simulink model "part2_2"  (R2018b)
settings: Solver=VariableStepAuto  StartTime=0.0  StopTime=10.0*0.1551  MaxStep=0.01*0.1551  RelTol=1e-3
settings Model: Creator=buddyugwumba1  LastModifiedBy=buddyugwumba1

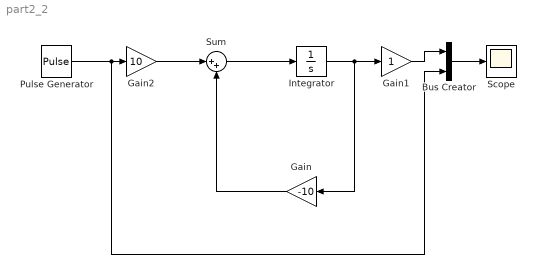
== system part2_2 ==
  Bus Creator : BusCreator  Inputs=2
  Gain : Gain  Gain=-10
  Gain1 : Gain
  Gain2 : Gain  Gain=10
  Integrator : Integrator
  Pulse Generator : DiscretePulseGenerator  PulseType=Time based  Period=20*0.1551  PulseWidth=99.99
  Scope : Scope
  Sum : Sum  Inputs=|++
  wires:
  Bus Creator/1 -> Scope/1
  Integrator/1 -> Gain/1, Gain1/1
  Gain1/1 -> Bus Creator/1
  Gain2/1 -> Sum/1
  Sum/1 -> Integrator/1
  Pulse Generator/1 -> Bus Creator/2, Gain2/1
  Gain/1 -> Sum/2
